simulink model "convert_temperatures"  (R2022b)
settings: Solver=VariableStepAuto  StartTime=0.0  StopTime=10.0  RelTol=1e-3
settings Model: Creator=Abanob_Sameh  LastModifiedBy=Abanob_Sameh

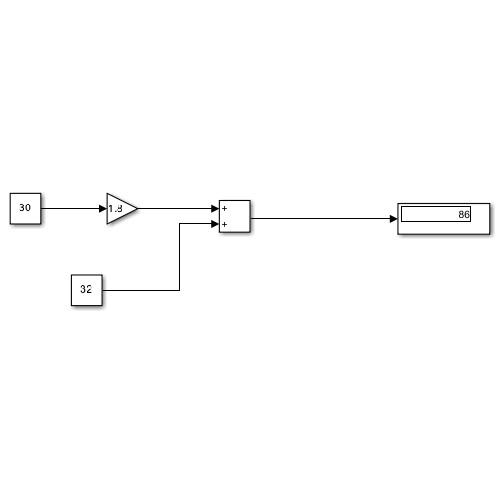
[thumbnail: Simulink's stored preview of the top-level diagram]
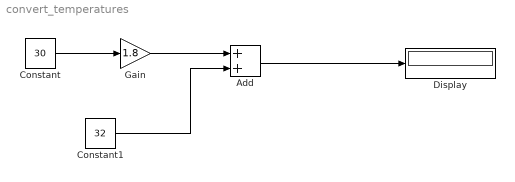
== system convert_temperatures ==
  Add : Sum
  Constant : Constant  Value=30
  Constant1 : Constant  Value=32
  Display : Display
  Gain : Gain  Gain=1.8
  wires:
  Add/1 -> Display/1
  Constant/1 -> Gain/1
  Constant1/1 -> Add/2
  Gain/1 -> Add/1
